simulink model "inverter"  (R2025a)
settings: Solver=ode4  StartTime=0.0  StopTime=1  FixedStep=1e-6  RelTol=1e-3
libraries: spsMosfetLib x4, simulink x4, spsSeriesRLCBranchLib x2, spsCurrentMeasurementLib x1, spsDCVoltageSourceLib x1, spsTriangleGeneratorLib x1, spsVoltageMeasurementLib x1, sps_lib x1
settings Model: Creator=Administrator  LastModifiedBy=ketan

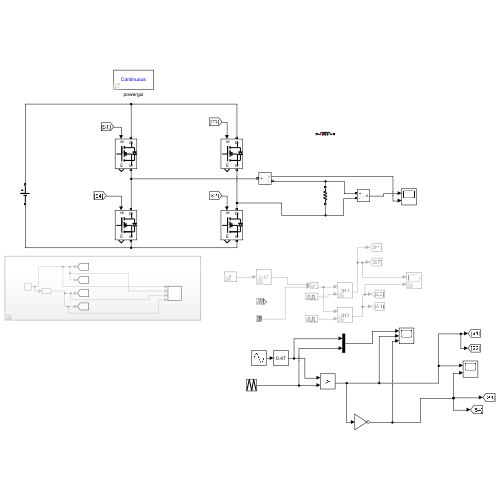
[thumbnail: Simulink's stored preview of the top-level diagram]
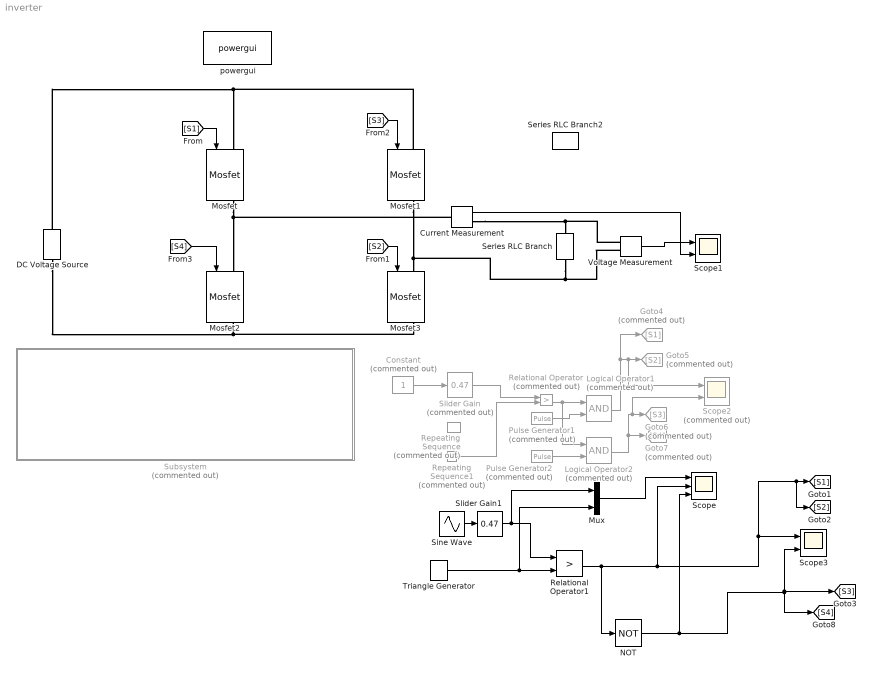
== system inverter ==
  Constant : Constant  Commented=on
  Current Measurement : spsCurrentMeasurementLib/Current Measurement  PhasorSimulation=off  OutputType=Complex  PSBequivalent=0
  DC Voltage Source : spsDCVoltageSourceLib/DC Voltage Source  Amplitude=350  Measurements=None
  Goto4 : Goto  Commented=on  GotoTag=S1
  Goto5 : Goto  Commented=on  GotoTag=S2
  Goto6 : Goto  Commented=on  GotoTag=S3
  Goto7 : Goto  Commented=on  GotoTag=S4
  Logical Operator1 : Logic  Commented=on  AllPortsSameDT=off  OutDataTypeStr=boolean
  Logical Operator2 : Logic  Commented=on  AllPortsSameDT=off  OutDataTypeStr=boolean
  Mosfet{,1..3} (4 alike) : spsMosfetLib/Mosfet  Ron=0.1  Lon=0  Rd=0.01  Vfd=0  IC=0  Rs=1e5  Cs=inf  Measurements=on
  Mux : Mux  Inputs=2
  NOT : Logic  Operator=NOT  IconShape=distinctive  AllPortsSameDT=off  OutDataTypeStr=boolean
  Pulse Generator1 : DiscretePulseGenerator  Commented=on  PulseType=Time based  Period=1/50  PulseWidth=50
  Pulse Generator2 : DiscretePulseGenerator  Commented=on  PulseType=Time based  Period=1/50  PulseWidth=50  PhaseDelay=0.01
  Relational Operator : RelationalOperator  Commented=on  Operator=>  OutDataTypeStr=boolean  RndMeth=Simplest  InputSameDT=off
  Relational Operator1 : RelationalOperator  Operator=>  OutDataTypeStr=boolean  RndMeth=Simplest  InputSameDT=off
  Repeating Sequence : simulink/Sources/Repeating Sequence  Commented=on  rep_seq_t=[0 1]*(1/100)  rep_seq_y=[0 1]
  Repeating Sequence1 : simulink/Sources/Repeating Sequence  Commented=on  rep_seq_t=[0 1]*(1/1000)  rep_seq_y=[0 1]
  Scope : Scope  NumInputPorts=3
      settings: ActiveDisplayYMinimum=-2.9754676070081043  ActiveDisplayYMaximum=6.2449368261935225  DataLoggingVariableName=ScopeData3
  Scope1 : Scope  NumInputPorts=2
      settings: TimeSpan=0.08  ActiveDisplayYMinimum=-428.92072760641645  ActiveDisplayYMaximum=428.92072760641645
  Scope2 : Scope  Commented=on  NumInputPorts=2
      settings: ActiveDisplayYMinimum=0.01137941305522272  ActiveDisplayYMaximum=1.0488645766571603  DataLoggingVariableName=ScopeData2
  Scope3 : Scope  NumInputPorts=2
      settings: ActiveDisplayYMinimum=-6.3040969699414511  ActiveDisplayYMaximum=4.8326513936097353  DataLoggingVariableName=ScopeData4
  Series RLC Branch : spsSeriesRLCBranchLib/Series RLC Branch  LConnTagsString=__new0  RConnTagsString=__new0  BranchType=R  Resistance=10  Inductance=1e-3  SetiL0=off  InitialCurrent=0  Capacitance=1e-6  Setx0=off  InitialVoltage=0  Measurements=None
  Series RLC Branch2 : spsSeriesRLCBranchLib/Series RLC Branch  LConnTagsString=__new0  RConnTagsString=__new0  BranchType=L  Resistance=10  Inductance=100e-3  SetiL0=off  InitialCurrent=0  Capacitance=1e-6  Setx0=off  InitialVoltage=0  Measurements=None
  Sine Wave : Sin  Amplitude=220  Frequency=2*pi*50  SampleTime=0
  Slider Gain : simulink/Math Operations/Slider Gain  Commented=on  gain=0.47  low=0  high=1
  Slider Gain1 : simulink/Math Operations/Slider Gain  gain=0.47  low=0  high=2
  Subsystem : Subsystem  Commented=on
  Triangle Generator : spsTriangleGeneratorLib/Triangle Generator  Freq=50  Phase=0  Ts=0
  Voltage Measurement : spsVoltageMeasurementLib/Voltage Measurement  PhasorSimulation=off  OutputType=Complex  PSBequivalent=0
  powergui : sps_lib/powergui  Priority=1  SimulationMode=Continuous  SampleTime=50e-6  frequency=60  Iterations=50  frequencyindice=0  Pbase=100e6  ErrMax=1e-4  UnitsV=kV  UnitsW=MW  buscounter=0  FunctionMessages=off  echomessages=off  EnableUseOfTLC=off  CurrentSourceSwitches=off  DisableSnubberDevices=off  DisableRonSwitches=off  DisableVfSwitches=off  DisplayEquations=off  AutomaticDiscreteSolvers=off  SolverType=Tustin/Backward Euler (TBE)  Interpol=off  ExternalGateDelay=off  methode=off  Ts=100  x0status=blocks  SPID=on  SwTol=0  HookPort=off  NonlinearTolerance=1e-4  nMaxIteration=100  ContinueOnMaxIteration=off  RestoreLinks=warning  ResistiveCurrentMeasurement=off  Frange=[0:2:500]  Ylog=off  Xlog=on  ShowGrid=off  save=off  variable=ZData  structure=0  ZoomFFT=off  StartTime=0.0  cycles=1  DisplayStyle=1  fundamental=60  FreqAxis=off  MaxFrequency=1000  frequencyindicesteady=1  RmsSteady=1  display=off
  wires:
  [S1] -> Mosfet/1
  [S2] -> Mosfet3/1
  [S3] -> Mosfet1/1
  [S4] -> Mosfet2/1
  Voltage Measurement/1 -> Scope1/1
  Current Measurement/1 -> Scope1/2
  Constant/1 -> Slider Gain/1
  Slider Gain/1 -> Relational Operator/1
  Logical Operator1/1 -> Scope2/1, Goto5/1, Goto4/1
  Relational Operator/1 -> Logical Operator2/1, Logical Operator1/1
  Pulse Generator1/1 -> Logical Operator1/2
  Logical Operator2/1 -> Goto7/1, Scope2/2, Goto6/1
  Pulse Generator2/1 -> Logical Operator2/2
  Repeating Sequence1/1 -> Relational Operator/2
  Mux/1 -> Scope/1
  Slider Gain1/1 -> Mux/1, Relational Operator1/1
  Sine Wave/1 -> Slider Gain1/1
  Triangle Generator/1 -> Mux/2, Relational Operator1/2
  Relational Operator1/1 -> NOT/1, Scope/2, Scope3/1, [S2], [S1]
  NOT/1 -> Scope/3, Scope3/2, [S3], [S4]
  connections:
  DC Voltage Source/RConn1 -- Mosfet/LConn1 -- Mosfet1/LConn1
  DC Voltage Source/LConn1 -- Mosfet3/RConn1 -- Mosfet2/RConn1
  Mosfet1/RConn1 -- Series RLC Branch/RConn1 -- Voltage Measurement/LConn2 -- Mosfet3/LConn1
  Mosfet/RConn1 -- Mosfet2/LConn1 -- Current Measurement/LConn1
  Voltage Measurement/LConn1 -- Current Measurement/RConn1 -- Series RLC Branch/LConn1

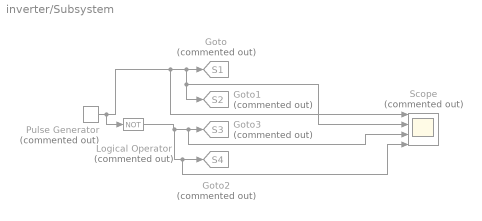
== system inverter/Subsystem ==
  Goto : Goto  Commented=on  GotoTag=S1  TagVisibility=global
  Goto1 : Goto  Commented=on  GotoTag=S2  TagVisibility=global
  Goto2 : Goto  Commented=on  GotoTag=S4  TagVisibility=global
  Goto3 : Goto  Commented=on  GotoTag=S3  TagVisibility=global
  Logical Operator : Logic  Commented=on  Operator=NOT  AllPortsSameDT=off  OutDataTypeStr=boolean
  Pulse Generator : DiscretePulseGenerator  Commented=on  PulseType=Time based  Period=1/50  PulseWidth=50
  Scope : Scope  Commented=on  NumInputPorts=4
      settings: ActiveDisplayYMinimum=-0.12499999999999997  ActiveDisplayYMaximum=1.125
  wires:
  Logical Operator/1 -> Scope/4, Goto2/1, Scope/3, Goto3/1
  Pulse Generator/1 -> Scope/1, Scope/2, Goto1/1, Goto/1, Logical Operator/1
